simulink model "model"  (R2012b)
settings: Solver=ode3  StartTime=0.0  StopTime=500  FixedStep=Ts  RelTol=1e-3
PreLoadFcn:
  | call
libraries: simulink x1
settings Model: Creator=shinm_000  LastModifiedBy=shinm_000
settings DataIOCC: SaveState=on

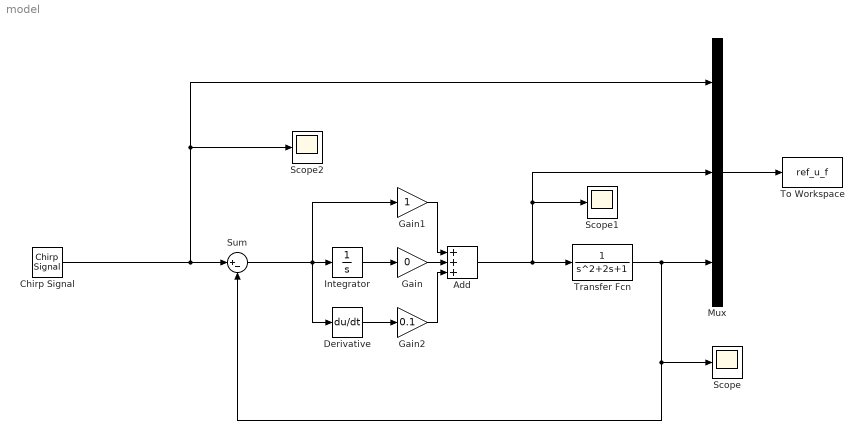
== system model ==
  Add : Sum  Inputs=+++
  Chirp Signal : simulink/Sources/Chirp Signal  f1=0.001  T=500  f2=0.2
  Derivative : Derivative
  Gain : Gain  Gain=0
  Gain1 : Gain
  Gain2 : Gain  Gain=0.1
  Integrator : Integrator
  Mux : Mux  Inputs=3
  Scope : Scope
      settings: TimeRange=40  YMin=0  YMax=1  MaxDataPoints=100000
  Scope1 : Scope
  Scope2 : Scope
      settings: SaveName=ScopeData2
  Sum : Sum  Inputs=|+-
  To Workspace : ToWorkspace  VariableName=ref_u_f  SampleTime=-1  SaveFormat=Timeseries
  Transfer Fcn : TransferFcn  Numerator=[0 0 1]
  wires:
  Chirp Signal/1 -> Mux/1, Scope2/1, Sum/1
  Transfer Fcn/1 -> Mux/3, Sum/2, Scope/1
  Integrator/1 -> Gain/1
  Gain1/1 -> Add/1
  Gain/1 -> Add/2
  Derivative/1 -> Gain2/1
  Gain2/1 -> Add/3
  Sum/1 -> Derivative/1, Gain1/1, Integrator/1
  Add/1 -> Transfer Fcn/1, Mux/2, Scope1/1
  Mux/1 -> To Workspace/1
